simulink model "single_phase_grid_connected_inverter"  (R2022b)
settings: Solver=FixedStepDiscrete  StartTime=0.0  StopTime=0.5  FixedStep=1e-6  RelTol=1e-3
libraries: spsSeriesRLCBranchLib x9, spsFourierLib x8, spsMosfetLib x4, spsCurrentMeasurementLib x3, simulink x3, spsVoltageMeasurementLib x3, spsMeanLib x2, spsRMSLib x2, spsDCVoltageSourceLib x1, spsIdealSwitchLib x1, spspowerguiLib x1, spsControlledVoltageSourceLib x1
(part 1 of 2)
settings Model: Creator=XIAO  LastModifiedBy=XIAO
settings SolverCC: AutoInsertRateTranBlk=on
settings DataIOCC: ReturnWorkspaceOutputs=off  LoggingToFile=on

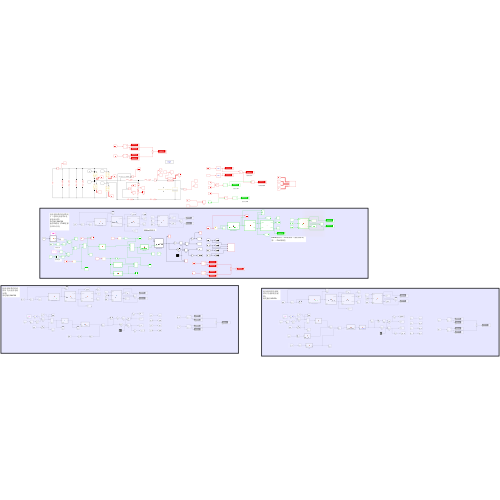
[thumbnail: Simulink's stored preview of the top-level diagram]
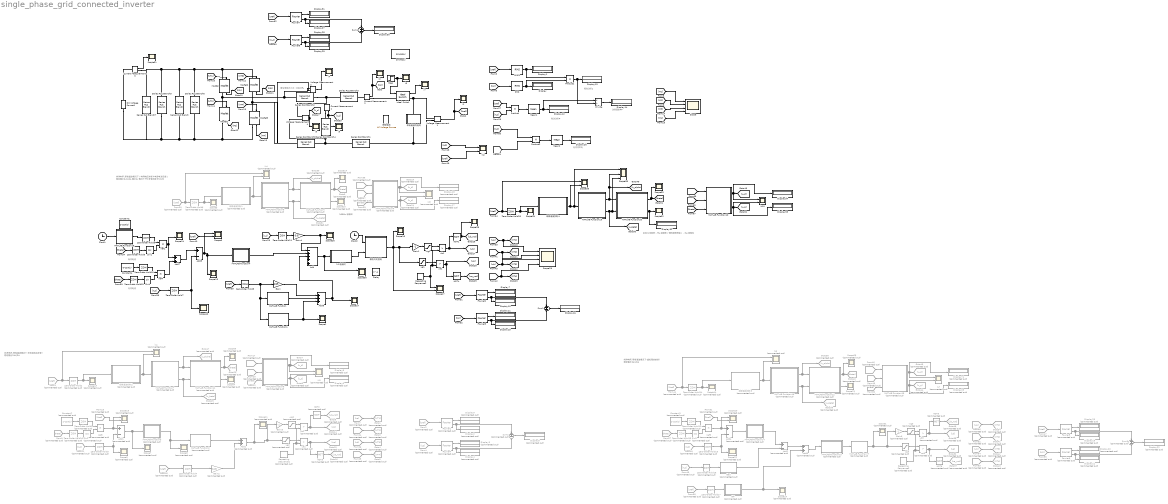
== system single_phase_grid_connected_inverter ==
  note: 100khz锁相环
  note: 视在功率s
  note: 寄生电阻大小为：R=2πfL
  note: 有功功率P
  note: 功率因数PF
  note: 纯净电网/带有谐波情况下（电网电压前馈+电容电流反馈）
      | 稳定输出24V/2A
      | 输出1A情况下THD任保持在5％以内
  note: 纯净电网/带有谐波情况下(无电容电流反馈)
      | 稳定输出24V/2A
  note: 纯净电网/带有谐波情况下(虚拟阻抗前馈)
      | 稳定输出24V/2A
  note: 无功功率Q
  note: 有功电流
  note: 无功电流
  note: 20khz锁相环，FLL锁频率（预防频率畸变），PLL锁相位
  -ug1 : Saturate  UpperLimit=1  LowerLimit=-1
  -ug2 : Saturate  Commented=on  UpperLimit=1  LowerLimit=-1
  -ug3 : Saturate  Commented=on  UpperLimit=1  LowerLimit=-1
  1.5倍延时 : MATLAB Function  TreatAsAtomicUnit=on
  Add : Sum  Inputs=-++++
  Add1 : Sum  Commented=on  Inputs=+-
  Add2 : Sum  Commented=on
  Add3 : Sum  Inputs=+-
  Add4 : Sum  Commented=on  Inputs=+-
  Add5 : Sum  Commented=on  Inputs=+-
  Add6 : Sum  Commented=on
  Add7 : Sum
  Add8 : Sum  Inputs=+++
  Clock1 : Clock
  Clock2 : Clock
  Constant1 : Constant  Value=2*sqrt(2)
  Constant2 : Constant  Commented=on  Value=2*sqrt(2)
  Constant3 : Constant  Commented=on  Value=2*sqrt(2)
  Constant4 : Constant  Value=0*sqrt(2)
  Current Measurement1 : spsCurrentMeasurementLib/Current Measurement  PhasorSimulation=off  OutputType=Complex  PSBequivalent=0
  Current Measurement2 : spsCurrentMeasurementLib/Current Measurement  PhasorSimulation=off  OutputType=Complex  PSBequivalent=0
  Current Measurement3 : spsCurrentMeasurementLib/Current Measurement  PhasorSimulation=off  OutputType=Complex  PSBequivalent=0
  DC Voltage Source1 : spsDCVoltageSourceLib/DC Voltage Source  Amplitude=45  Measurements=None
  Delay : Delay  DelayLength=1  SampleTime=5e-5
  Display{,1,7,10..16,26..34} (19 alike) : Display
  Display{2..6,8..9,17..25} (16 alike) : Display  Commented=on
  Divide : Product  Inputs=*/
  Fourier{1,4..6} (4 alike) : spsFourierLib/Fourier  Commented=on  Freq=50  n=1  InInit=[0, 0]  Ts=1e-6
  Fourier{2..3,7..8} (4 alike) : spsFourierLib/Fourier  Freq=50  n=1  InInit=[0, 0]  Ts=1e-6
  From{1..2,16,23,30,44,47,51,58} (9 alike) : From  Commented=on  GotoTag=Uref
  From17 : From  Commented=on  GotoTag=u_alpha
  From20 : From  Commented=on  GotoTag=u_beta
  From{4,21,45,49,55} (5 alike) : From  Commented=on  GotoTag=IL2
  From{9,22,39,50,57} (5 alike) : From  Commented=on  GotoTag=theta
  From24 : From  Commented=on  GotoTag=ua_not
  From25 : From  Commented=on  GotoTag=ub_not
  From26 : From  Commented=on  GotoTag=ub
  From36 : From  Commented=on  GotoTag=u_alpha
  From37 : From  Commented=on  GotoTag=u_beta
  From46 : From  Commented=on  GotoTag=u_alpha
  From48 : From  Commented=on  GotoTag=u_beta
  From52 : From  Commented=on  GotoTag=ua_not
  From53 : From  Commented=on  GotoTag=ub_not
  From54 : From  Commented=on  GotoTag=ub
  From56 : From  Commented=on  GotoTag=ua
  From7 : From  Commented=on  GotoTag=ua
  Gad : MATLAB Function  Commented=on  TreatAsAtomicUnit=on
  Gain : Gain  Gain=1/45
  Gain1 : Gain  Gain=-1
  Gain2 : Gain  Commented=on  Gain=1/45
  Gain3 : Gain  Commented=on  Gain=-1
  Gain4 : Gain  Gain=0.07
  Gain6 : Gain  Commented=on  Gain=-1
  Gff : MATLAB Function  Commented=on  TreatAsAtomicUnit=on
  Goto1 : Goto  Commented=on  GotoTag=VT1
  Goto14 : Goto  Commented=on  GotoTag=ub
  Goto15 : Goto  Commented=on  GotoTag=ua
  Goto16 : Goto  Commented=on  GotoTag=ua_not
  Goto17 : Goto  Commented=on  GotoTag=u_alpha
  Goto19 : Goto  Commented=on  GotoTag=u_beta
  Goto20 : Goto  Commented=on  GotoTag=theta
  Goto24 : Goto  Commented=on  GotoTag=u_q
  Goto25 : Goto  Commented=on  GotoTag=u_d
  Goto3 : Goto  Commented=on  GotoTag=VT2
  Goto30 : Goto  Commented=on  GotoTag=u_alpha
  Goto31 : Goto  Commented=on  GotoTag=u_beta
  Goto34 : Goto  Commented=on  GotoTag=VT1
  Goto35 : Goto  Commented=on  GotoTag=ub
  Goto36 : Goto  Commented=on  GotoTag=ua
  Goto37 : Goto  Commented=on  GotoTag=ua_not
  Goto38 : Goto  Commented=on  GotoTag=u_alpha
  Goto39 : Goto  Commented=on  GotoTag=u_beta
  Goto4 : Goto  Commented=on  GotoTag=VT3
  Goto40 : Goto  Commented=on  GotoTag=theta
  Goto41 : Goto  Commented=on  GotoTag=VT2
  Goto42 : Goto  Commented=on  GotoTag=VT3
  Goto43 : Goto  Commented=on  GotoTag=VT4
  Goto44 : Goto  Commented=on  GotoTag=u_q
  Goto45 : Goto  Commented=on  GotoTag=u_d
  Goto46 : Goto  Commented=on  GotoTag=ub_not
  Goto5 : Goto  Commented=on  GotoTag=VT4
  Goto6 : Goto  Commented=on  GotoTag=u_q
  Goto7 : Goto  Commented=on  GotoTag=u_d
  Goto8 : Goto  Commented=on  GotoTag=ub_not
  Goto9 : Goto  Commented=on  GotoTag=theta
  Ideal Switch : spsIdealSwitchLib/Ideal Switch  Ron=0.001  Lon=0  IC=0  Rs=1e5  Cs=inf  Measurements=on
  Iref1 : Product
  Iref2 : Product  Commented=on
  Iref3 : Product  Commented=on
  Iref4 : Product
  MATLAB Function : MATLAB Function  TreatAsAtomicUnit=on
  MATLAB Function1 : MATLAB Function  TreatAsAtomicUnit=on
  MATLAB Function10 : MATLAB Function  TreatAsAtomicUnit=on
  MATLAB Function11 : MATLAB Function  Commented=on  TreatAsAtomicUnit=on
  MATLAB Function12 : MATLAB Function  Commented=on  TreatAsAtomicUnit=on
  MATLAB Function13 : MATLAB Function  Commented=on  TreatAsAtomicUnit=on
  MATLAB Function14 : MATLAB Function  Commented=on  TreatAsAtomicUnit=on
  MATLAB Function15 : MATLAB Function  Commented=on  TreatAsAtomicUnit=on
  MATLAB Function16 : MATLAB Function  Commented=on  TreatAsAtomicUnit=on
  MATLAB Function17 : MATLAB Function  Commented=on  TreatAsAtomicUnit=on
  MATLAB Function18 : MATLAB Function  TreatAsAtomicUnit=on
  MATLAB Function19 : MATLAB Function  TreatAsAtomicUnit=on
  MATLAB Function2 : MATLAB Function  Commented=on  TreatAsAtomicUnit=on
  MATLAB Function20 : MATLAB Function  TreatAsAtomicUnit=on
  MATLAB Function3 : MATLAB Function  Commented=on  TreatAsAtomicUnit=on
  MATLAB Function4 : MATLAB Function  TreatAsAtomicUnit=on
  MATLAB Function5 : MATLAB Function  Commented=on  TreatAsAtomicUnit=on
  MATLAB Function6 : MATLAB Function  Commented=on  TreatAsAtomicUnit=on
  MATLAB Function7 : MATLAB Function  Commented=on  TreatAsAtomicUnit=on
  MATLAB Function8 : MATLAB Function  Commented=on  TreatAsAtomicUnit=on
  MATLAB Function9 : MATLAB Function  Commented=on  TreatAsAtomicUnit=on
  Mean1 : spsMeanLib/Mean  Freq=50  Vinit=0  Ts=5e-5
  Mean2 : spsMeanLib/Mean  Freq=50  Vinit=0  Ts=5e-5
  Mosfet{,1..3} (4 alike) : spsMosfetLib/Mosfet  Ron=0.1  Lon=0  Rd=0.01  Vfd=0  IC=0  Rs=1e5  Cs=inf  Measurements=on
  NOT1 : Logic  Operator=NOT  IconShape=distinctive  AllPortsSameDT=off  OutDataTypeStr=boolean
  NOT{2..3,5..6} (4 alike) : Logic  Commented=on  Operator=NOT  IconShape=distinctive  AllPortsSameDT=off  OutDataTypeStr=boolean
  NOT4 : Logic  Operator=NOT  IconShape=distinctive  AllPortsSameDT=off  OutDataTypeStr=boolean
  Product : Product
  Product1 : Product
  Product2 : Product
  RMS : spsRMSLib/RMS  TrueRMS=on  Freq=50  RMSInit=24  Ts=1e-6
  RMS1 : spsRMSLib/RMS  TrueRMS=on  Freq=50  RMSInit=24  Ts=1e-6
  Repeating Sequence1 : simulink/Sources/Repeating Sequence  Commented=on  rep_seq_t=[0, 5e-5, 1e-4]  rep_seq_y=[-1, 1, -1]
  Repeating Sequence2 : simulink/Sources/Repeating Sequence  rep_seq_t=[0, 5e-5, 1e-4]  rep_seq_y=[-1, 1, -1]
  Repeating Sequence3 : simulink/Sources/Repeating Sequence  Commented=on  rep_seq_t=[0, 5e-5, 1e-4]  rep_seq_y=[-1, 1, -1]
  Scope : Scope  NumInputPorts=4
  Scope{1,12..13,16,26..28,31..34} (11 alike) : Scope
  Scope{2..5,7..11,14..15,18,21..22,25} (15 alike) : Scope  Commented=on
  Scope{6,17,24,30,35} (5 alike) : Scope  NumInputPorts=2
  Scope19 : Scope  Commented=on  NumInputPorts=2
  Scope20 : Scope  Commented=on  NumInputPorts=2
  Scope23 : Scope  Commented=on  NumInputPorts=2
  Scope29 : Scope  NumInputPorts=4
  Scope36 : Scope  NumInputPorts=3
  Series RLC Branch{,5..7} (4 alike) : spsSeriesRLCBranchLib/Series RLC Branch  LConnTagsString=__new0  RConnTagsString=__new0  BranchType=RC  Resistance=0.01  Inductance=0  SetiL0=off  InitialCurrent=0  Capacitance=470e-6  Setx0=off  InitialVoltage=0  Measurements=None
  Series RLC Branch1 : spsSeriesRLCBranchLib/Series RLC Branch  LConnTagsString=__new0  RConnTagsString=__new0  BranchType=RL  Resistance=0.1  Inductance=0.00012  SetiL0=off  InitialCurrent=0  Capacitance=220e-6  Setx0=off  InitialVoltage=0  Measurements=None
  Series RLC Branch2 : spsSeriesRLCBranchLib/Series RLC Branch  LConnTagsString=__new0  RConnTagsString=__new0  BranchType=RL  Resistance=0.1  Inductance=0.0015  SetiL0=off  InitialCurrent=0  Capacitance=220e-6  Setx0=off  InitialVoltage=0  Measurements=None
  Series RLC Branch3 : spsSeriesRLCBranchLib/Series RLC Branch  LConnTagsString=__new0  RConnTagsString=__new0  BranchType=RL  Resistance=0.1  Inductance=0.00012  SetiL0=off  InitialCurrent=0  Capacitance=220e-6  Setx0=off  InitialVoltage=0  Measurements=None
  Series RLC Branch4 : spsSeriesRLCBranchLib/Series RLC Branch  LConnTagsString=__new0  RConnTagsString=__new0  BranchType=RC  Resistance=0.1  Inductance=0  SetiL0=off  InitialCurrent=0  Capacitance=10e-6  Setx0=off  InitialVoltage=0  Measurements=None
  Series RLC Branch8 : spsSeriesRLCBranchLib/Series RLC Branch  LConnTagsString=__new0  RConnTagsString=__new0  BranchType=RL  Resistance=0.1  Inductance=0.0015  SetiL0=off  InitialCurrent=0  Capacitance=220e-6  Setx0=off  InitialVoltage=0  Measurements=None
  Sin1 : Trigonometry  Operator=cos
  Sin2 : Trigonometry  Commented=on  Operator=cos
  Sin3 : Trigonometry  Commented=on  Operator=cos
  Sin4 : Trigonometry
  Step : Step  Time=0.25  SampleTime=1e-6
  Sum1 : Sum  Inputs=+-
  Sum2 : Sum  Commented=on  Inputs=+-
  Sum3 : Sum  Commented=on  Inputs=+-
  Sum4 : Sum  Inputs=+-
  Voltage Measurement1 : spsVoltageMeasurementLib/Voltage Measurement  PhasorSimulation=off  OutputType=Complex  PSBequivalent=0
  Voltage Measurement2 : spsVoltageMeasurementLib/Voltage Measurement  PhasorSimulation=off  OutputType=Complex  PSBequivalent=0
  Voltage Measurement4 : spsVoltageMeasurementLib/Voltage Measurement  PhasorSimulation=off  OutputType=Complex  PSBequivalent=0
  Zero-Order Hold{1,3..4,10,12..13,15..17} (9 alike) : ZeroOrderHold  Commented=on  SampleTime=5e-5
  Zero-Order Hold{5,7..9,11,18..20} (8 alike) : ZeroOrderHold  SampleTime=5e-5
  Zero-Order Hold14 : ZeroOrderHold  Commented=on  SampleTime=1e-5
  Zero-Order Hold2 : ZeroOrderHold  Commented=on  SampleTime=1e-5
  Zero-Order Hold6 : ZeroOrderHold  Commented=on  SampleTime=1e-5
  i{1..7} (7 alike) : Scope
  iL{1,3..7} (6 alike) : Scope  Commented=on  NumInputPorts=2
  iL10 : Scope  NumInputPorts=2
  iL2 : Scope  NumInputPorts=2
  powergui : spspowerguiLib/powergui  Priority=1  SimulationMode=Discrete  SampleTime=1e-6  frequency=60  Iterations=50  frequencyindice=0  Pbase=100e6  ErrMax=1e-4  UnitsV=kV  UnitsW=MW  buscounter=0  FunctionMessages=off  echomessages=off  EnableUseOfTLC=off  CurrentSourceSwitches=off  DisableSnubberDevices=off  DisableRonSwitches=off  DisableVfSwitches=off  DisplayEquations=off  AutomaticDiscreteSolvers=off  SolverType=Tustin/Backward Euler (TBE)  Interpol=off  ExternalGateDelay=off  methode=off  Ts=100  x0status=blocks  SPID=on  SwTol=0  HookPort=off  NonlinearTolerance=1e-4  nMaxIteration=100  ContinueOnMaxIteration=off  RestoreLinks=warning  ResistiveCurrentMeasurement=off  Frange=[0:2:500]  Ylog=off  Xlog=on  ShowGrid=off  save=off  variable=ZData  structure=0  ZoomFFT=off  StartTime=0.0  cycles=1  DisplayStyle=1  fundamental=60  FreqAxis=off  MaxFrequency=1000  frequencyindicesteady=1  RmsSteady=1  display=off
  ua1 : RelationalOperator  Operator=>  OutDataTypeStr=boolean  RndMeth=Simplest  InputSameDT=off
  ua2 : RelationalOperator  Commented=on  Operator=>  OutDataTypeStr=boolean  RndMeth=Simplest  InputSameDT=off
  ua3 : RelationalOperator  Commented=on  Operator=>  OutDataTypeStr=boolean  RndMeth=Simplest  InputSameDT=off
  ub1 : RelationalOperator  Operator=>  OutDataTypeStr=boolean  RndMeth=Simplest  InputSameDT=off
  ub2 : RelationalOperator  Commented=on  Operator=>  OutDataTypeStr=boolean  RndMeth=Simplest  InputSameDT=off
  ub3 : RelationalOperator  Commented=on  Operator=>  OutDataTypeStr=boolean  RndMeth=Simplest  InputSameDT=off
  ug1 : Saturate  UpperLimit=1  LowerLimit=-1
  ug2 : Saturate  Commented=on  UpperLimit=1  LowerLimit=-1
  ug3 : Saturate  Commented=on  UpperLimit=1  LowerLimit=-1
  带有谐波的电网 : Subsystem
  模仿开关控制 : MATLAB Function  TreatAsAtomicUnit=on
  理想电网 : spsACVoltageSourceLib/AC Voltage Source  Amplitude=24*1.414  Phase=0  Frequency=50  SampleTime=0  Measurements=None  BusType=swing  Pref=10e3  Qref=0  Qmin=-inf  Qmax=+inf
  级联谐波抑制1 : MATLAB Function  Commented=on  TreatAsAtomicUnit=on
  级联谐波抑制2 : MATLAB Function  Commented=on  TreatAsAtomicUnit=on
  级联谐波抑制3 : MATLAB Function  Commented=on  TreatAsAtomicUnit=on
  级联谐波抑制4 : MATLAB Function  TreatAsAtomicUnit=on
  wires:
  [IL2] -> RMS/1
  [VT3] -> Mosfet2/1
  RMS/1 -> Product1/2, Display/1
  Mosfet3/1 -> [M4]
  [M3] -> Scope/3
  [Uref] -> RMS1/1
  Mosfet1/1 -> [M2]
  [VT2] -> Mosfet1/1
  [M2] -> Scope/2
  [VT4] -> Mosfet3/1
  [M4] -> Scope/4
  [VT1] -> Mosfet/1
  Mosfet/1 -> [M1]
  RMS1/1 -> Product1/1, Display1/1
  Mosfet2/1 -> [M3]
  [M1] -> Scope/1
  Voltage Measurement1/1 -> i1/1, [Uref]
  [IL2] -> iL2/1
  [Uref] -> iL2/2
  Current Measurement2/1 -> [IL2], i2/1
  Voltage Measurement2/1 -> i4/1
  [Uref] -> Product/1
  [IL2] -> Product/2
  Product/1 -> Mean1/1
  Mean1/1 -> Divide/1, Display12/1
  Product1/1 -> Divide/2, Display13/1
  Divide/1 -> Display14/1
  [IL2] -> Zero-Order Hold7/1
  Zero-Order Hold9/1 -> Sin1/1
  MATLAB Function9/2(qerror) -> Scope10/1
  [Uref] -> Scope6/2
  级联谐波抑制1/1(y) -> iL4/2, MATLAB Function8/1(U_in)
  Zero-Order Hold8/1 -> MATLAB Function1/1(u), MATLAB Function/1(u), Gain/1
  MATLAB Function9/1(theta) -> Scope15/1, Goto9/1
  MATLAB Function5/2(q) -> Display17/1, Goto24/1, iL5/2
  Fourier3/1 -> Display11/1
  [ua_not] -> Scope29/2, [VT2]
  [ub] -> Scope29/3, [VT3]
  Fourier3/2 -> Sum1/2, Display15/1
  [ub_not] -> Scope29/4, [VT4]
  -ug1/1 -> ub1/1
  ug1/1 -> ua1/1
  Sum1/1 -> Display16/1
  Fourier2/2 -> Display10/1, Sum1/1
  MATLAB Function8/2(deltaU_prime) -> Goto31/1, MATLAB Function9/2(u_beta)
  [IL2] -> Fourier3/1
  [Uref] -> Fourier2/1
  [Uref] -> Zero-Order Hold8/1
  Zero-Order Hold6/1 -> 级联谐波抑制1/1(u), Scope3/1
  From36/1 -> MATLAB Function5/1(alpha)
  [ua] -> Scope29/1, [VT1]
  ub1/1 -> [ub], NOT1/1
  Gain1/1 -> -ug1/1
  ua1/1 -> [ua], NOT4/1
  MATLAB Function5/1(d) -> iL5/1, Display18/1, Goto25/1
  NOT4/1 -> [ua_not]
  Sin1/1 -> Iref1/2
  MATLAB Function8/1(U_prime) -> MATLAB Function9/1(u_alpha), Goto30/1
  From30/1 -> iL4/1, Zero-Order Hold6/1
  From39/1 -> MATLAB Function5/3(theta)
  Fourier2/1 -> Display7/1
  [theta] -> Zero-Order Hold9/1
  From37/1 -> MATLAB Function5/2(beta)
  NOT1/1 -> Scope28/1, [ub_not]
  Zero-Order Hold5/1 -> Iref1/1
  Zero-Order Hold7/1 -> Add3/2, Scope12/1
  MATLAB Function3/1(y) -> MATLAB Function2/1(u), Scope8/1
  MATLAB Function7/1(U_prime) -> MATLAB Function11/1(u_alpha), Goto17/1
  Sin2/1 -> Iref2/2
  Iref2/1 -> Scope19/1, Add1/1
  NOT3/1 -> Goto16/1
  MATLAB Function6/1(d) -> iL3/1, Display8/1, Goto7/1
  ub2/1 -> Goto14/1, NOT2/1
  Gain3/1 -> -ug2/1
  From7/1 -> Goto1/1
  From2/1 -> Fourier1/1
  From17/1 -> MATLAB Function6/1(alpha)
  From16/1 -> Zero-Order Hold4/1
  From4/1 -> Fourier4/1
  From22/1 -> MATLAB Function6/3(theta)
  级联谐波抑制2/1(y) -> iL1/2, MATLAB Function7/1(U_in)
  Sum2/1 -> Display5/1
  ug2/1 -> ua2/1
  Zero-Order Hold4/1 -> Gain2/1
  From1/1 -> iL1/1, Zero-Order Hold2/1
  -ug2/1 -> ub2/1
  Fourier1/1 -> Display9/1
  Fourier4/2 -> Sum2/2, Display4/1
  Fourier1/2 -> Display2/1, Sum2/1
  From25/1 -> Goto5/1
  From26/1 -> Goto4/1
  ua2/1 -> Goto15/1, NOT3/1
  From24/1 -> Goto3/1
  MATLAB Function11/1(theta) -> Scope9/1, Goto20/1
  Repeating Sequence1/1 -> ub2/2, ua2/2
  From9/1 -> Zero-Order Hold10/1
  Fourier4/1 -> Display3/1
  Zero-Order Hold1/1 -> Iref2/1
  MATLAB Function6/2(q) -> Display6/1, Goto6/1, iL3/2
  From20/1 -> MATLAB Function6/2(beta)
  Constant2/1 -> Zero-Order Hold1/1
  MATLAB Function11/2(qerror) -> Scope4/1
  Zero-Order Hold10/1 -> Sin2/1
  MATLAB Function7/2(deltaU_prime) -> Goto19/1, MATLAB Function11/2(u_beta)
  NOT2/1 -> Goto8/1
  From21/1 -> Zero-Order Hold3/1
  Zero-Order Hold2/1 -> 级联谐波抑制2/1(u), Scope18/1
  From23/1 -> Scope19/2
  Add1/1 -> MATLAB Function3/1(u), Scope7/1
  Zero-Order Hold3/1 -> Add1/2, Scope5/1
  Current Measurement1/1 -> [I_c], i3/1
  [I_c] -> Zero-Order Hold11/1
  Zero-Order Hold11/1 -> Gain4/1
  Add2/1 -> Scope11/1, Gain3/1, ug2/1
  Gain2/1 -> Add2/2
  Gain4/1 -> Scope26/1, Add/1
  MATLAB Function/1(y) -> Add8/2
  Fourier6/2 -> Sum3/2, Display21/1
  Fourier5/1 -> Display25/1
  -ug3/1 -> ub3/1
  From44/1 -> iL6/1, Zero-Order Hold14/1
  Zero-Order Hold15/1 -> Add4/2, Scope22/1
  From51/1 -> Scope20/2
  NOT5/1 -> Goto46/1
  From49/1 -> Zero-Order Hold15/1
  MATLAB Function16/2(deltaU_prime) -> Goto39/1, MATLAB Function12/2(u_beta)
  Zero-Order Hold14/1 -> 级联谐波抑制3/1(u), Scope14/1
  Zero-Order Hold13/1 -> Sin3/1
  Constant3/1 -> Zero-Order Hold12/1
  From57/1 -> Zero-Order Hold13/1
  MATLAB Function12/2(qerror) -> Scope21/1
  Fourier5/2 -> Display19/1, Sum3/1
  From52/1 -> Goto41/1
  MATLAB Function12/1(theta) -> Scope25/1, Goto40/1
  From48/1 -> MATLAB Function15/2(beta)
  ua3/1 -> Goto36/1, NOT6/1
  Repeating Sequence3/1 -> ub3/2, ua3/2
  Iref3/1 -> Scope20/1, Add4/1
  Zero-Order Hold12/1 -> Iref3/1
  Sin3/1 -> Iref3/2
  NOT6/1 -> Goto37/1
  Sum3/1 -> Display22/1
  MATLAB Function16/1(U_prime) -> MATLAB Function12/1(u_alpha), Goto38/1
  级联谐波抑制3/1(y) -> iL6/2, MATLAB Function16/1(U_in)
  From50/1 -> MATLAB Function15/3(theta)
  From55/1 -> Fourier6/1
  From46/1 -> MATLAB Function15/1(alpha)
  From47/1 -> Fourier5/1
  From56/1 -> Goto34/1
  Gain6/1 -> -ug3/1
  Add4/1 -> MATLAB Function14/1(u)
  ub3/1 -> Goto35/1, NOT5/1
  MATLAB Function15/1(d) -> iL7/1, Display24/1, Goto45/1
  ug3/1 -> ua3/1
  MATLAB Function15/2(q) -> Display23/1, Goto44/1, iL7/2
  From53/1 -> Goto43/1
  From54/1 -> Goto42/1
  Fourier6/1 -> Display20/1
  MATLAB Function14/1(y) -> Add5/1
  From45/1 -> Zero-Order Hold16/1
  Zero-Order Hold16/1 -> Gad/1(u)
  Gff/1(y) -> Scope23/1, Add6/2
  Zero-Order Hold17/1 -> Gff/1(u)
  From58/1 -> Zero-Order Hold17/1
  MATLAB Function2/1(y) -> Add2/1
  MATLAB Function13/1(y) -> MATLAB Function17/1(u)
  Gain/1 -> Add8/1
  MATLAB Function1/1(y) -> Add8/3, Scope1/1
  MATLAB Function17/1(y) -> Gain6/1, ug3/1, Scope2/1
  Gad/1(y) -> Add5/2
  Add5/1 -> Add6/1
  Add6/1 -> MATLAB Function13/1(u)
  Sin4/1 -> Iref4/2
  [theta] -> Zero-Order Hold19/1
  Zero-Order Hold18/1 -> Iref4/1
  Constant4/1 -> Zero-Order Hold18/1
  Zero-Order Hold19/1 -> Sin4/1
  Iref1/1 -> Add7/1, Scope24/2
  Iref4/1 -> Add7/2
  Add7/1 -> Add3/1
  [IL2] -> Product2/1
  Product2/1 -> Mean2/1
  Mean2/1 -> Display26/1
  [u_beta] -> Product2/2
  Add3/1 -> Scope6/1, MATLAB Function4/1(u), Scope13/1
  Voltage Measurement4/1 -> i5/1, [V_c]
  Step/1 -> Ideal Switch/1, i6/1
  Ideal Switch/1 -> i7/1
  Clock1/1 -> MATLAB Function18/1(t)
  MATLAB Function18/1(I_amp) -> Zero-Order Hold5/1
  Add8/1 -> Add/3, Scope27/1
  Fourier7/2 -> Display27/1, Sum4/1
  [Uref] -> Fourier7/1
  Fourier7/1 -> Display31/1
  Sum4/1 -> Display30/1
  Fourier8/1 -> Display28/1
  Fourier8/2 -> Sum4/2, Display29/1
  [V_c] -> Fourier8/1
  模仿开关控制/1(mod_out) -> Scope16/1, Gain1/1, ug1/1, Scope17/2
  Clock2/1 -> 模仿开关控制/1(t)
  Repeating Sequence2/1 -> ub1/2, ua1/2, Scope17/1
  MATLAB Function4/1(y) -> Add/2
  Add/1 -> 1.5倍延时/1(u), Scope30/1
  1.5倍延时/1(y) -> 模仿开关控制/2(mod_in)
  Current Measurement3/1 -> Scope31/1
  级联谐波抑制4/1(y) -> Scope35/2, Scope36/1, MATLAB Function19/1(uin)
  [u_beta] -> MATLAB Function10/2(beta)
  [Uref] -> Scope35/1, Zero-Order Hold20/1
  MATLAB Function20/2(qerror) -> Scope32/1, Display32/1
  [u_alpha] -> MATLAB Function10/1(alpha)
  Zero-Order Hold20/1 -> 级联谐波抑制4/1(u), Scope34/1
  MATLAB Function20/1(theta) -> Scope33/1, [theta]
  MATLAB Function10/1(d) -> iL10/1, Display34/1, [u_d]
  [theta] -> MATLAB Function10/3(theta)
  MATLAB Function10/2(q) -> Display33/1, [u_q], iL10/2
  MATLAB Function19/1(alpha) -> Scope36/2, [u_alpha], MATLAB Function20/1(u_alpha)
  MATLAB Function19/2(beta) -> Scope36/3, MATLAB Function20/2(u_beta), [u_beta]
  connections:
  Mosfet1/RConn1 -- DC Voltage Source1/LConn1 -- Series RLC Branch7/RConn1 -- Series RLC Branch5/RConn1 -- Series RLC Branch/RConn1 -- Series RLC Branch6/RConn1 -- Mosfet3/RConn1
  Mosfet/LConn1 -- Current Measurement3/RConn1 -- Series RLC Branch7/LConn1 -- Series RLC Branch5/LConn1 -- Series RLC Branch/LConn1 -- Series RLC Branch6/LConn1 -- Mosfet2/LConn1
  Series RLC Branch2/RConn1 -- Voltage Measurement2/LConn1 -- Mosfet/RConn1 -- Mosfet1/LConn1
  Mosfet3/LConn1 -- Series RLC Branch8/RConn1 -- Voltage Measurement2/LConn2 -- Mosfet2/RConn1
  Series RLC Branch2/LConn1 -- Current Measurement1/LConn1 -- Voltage Measurement4/LConn1 -- Series RLC Branch3/RConn1
  Current Measurement2/LConn1 -- Series RLC Branch3/LConn1
  带有谐波的电网/RConn1 -- Voltage Measurement1/LConn1 -- Ideal Switch/RConn1
  Current Measurement1/RConn1 -- Series RLC Branch4/LConn1
  Current Measurement2/RConn1 -- Ideal Switch/LConn1
  Current Measurement3/LConn1 -- DC Voltage Source1/RConn1
  Voltage Measurement1/LConn2 -- 带有谐波的电网/LConn1 -- Series RLC Branch1/LConn1
  Series RLC Branch4/RConn1 -- Series RLC Branch8/LConn1 -- Series RLC Branch1/RConn1 -- Voltage Measurement4/LConn2

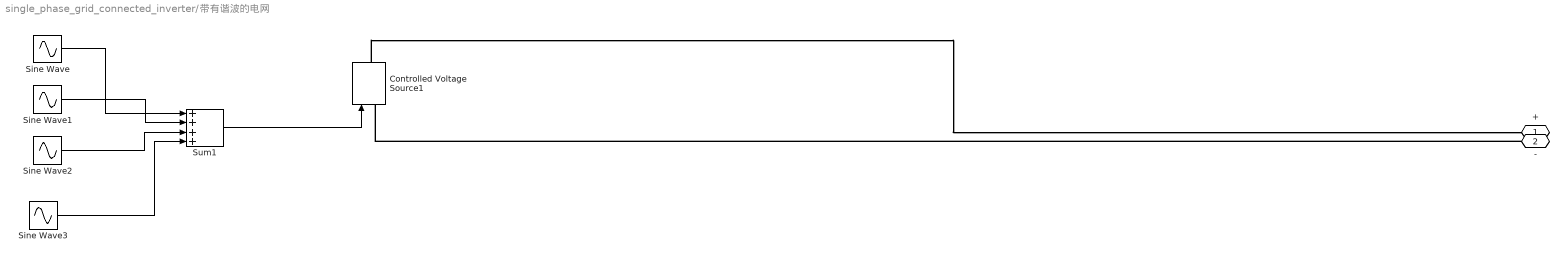
== system single_phase_grid_connected_inverter/带有谐波的电网 ==
  Controlled Voltage Source1 : spsControlledVoltageSourceLib/Controlled Voltage Source  Initialize=off  Source_Type=AC  Amplitude=0  Phase=0  Frequency=0  Measurements=Voltage
  Sine Wave : Sin  Amplitude=24*sqrt(2)  Frequency=100*pi  SampleTime=0
  Sine Wave1 : Sin  Amplitude=0.04*24*sqrt(2)  Frequency=300*pi  SampleTime=0
  Sine Wave2 : Sin  Amplitude=0.03*24*sqrt(2)  Frequency=500*pi  SampleTime=0
  Sine Wave3 : Sin  Amplitude=0.02*24*sqrt(2)  Frequency=700*pi  SampleTime=0
  Sum1 : Sum  Inputs=++++
  + : PMIOPort  Side=Right
  - : PMIOPort  Port=2  Side=Left
  wires:
  Sum1/1 -> Controlled Voltage Source1/1
  Sine Wave1/1 -> Sum1/2
  Sine Wave/1 -> Sum1/1
  Sine Wave3/1 -> Sum1/4
  Sine Wave2/1 -> Sum1/3
  connections:
  -/RConn1 -- Controlled Voltage Source1/LConn1
  Controlled Voltage Source1/RConn1 -- +/RConn1

== matlab function single_phase_grid_connected_inverter/MATLAB Function9 ==
  data: u_alpha input; theta output; u_beta input; qerror output
function [theta, qerror] = SRF_PLL(u_alpha, u_beta)
% 同步旋转坐标系锁相环 SRF-PLL（严格匹配框图逻辑）
% 输入
%   u_alpha:  α轴输入信号（对应框图的v'，与电网电压同相）
%   u_beta:   β轴输入信号（对应框图的qv'，与电网电压正交90°）
% 输出
%   theta:    锁相得到的电网相位 [0, 2π)
%   qerror:   q轴相位误差（锁相锁定时趋近于0）
% 适配：仿真步长 Ts=1e-5（10kHz采样），基波频率50Hz

    %% ===================== 1. 固定参数配置 =====================
    Ts = 1e-5;               % 采样时间，必须与全局仿真步长完全一致
    f0 = 50;                  % 电网额定基波频率 (Hz)
    w0 = 2 * pi * f0;        % 额定角频率 (rad/s)
    
    % PI控制器参数（适配10kHz采样，可按需调整）
    kp_pll = 60;              % 比例系数：增大加快锁相响应，过大易振荡
    ki_pll = 5000;            % 积分系数：增大减小稳态相位误差，过大影响稳定性

    %% ===================== 2. 持久变量初始化（仅首次运行执行） =====================
    persistent theta_prev     % 上一拍的锁相相位
    persistent xi_pll         % PI控制器的积分项（抗饱和）
    
    if isempty(theta_prev)
        theta_prev = 0;       % 相位初始值清零
        xi_pll = 0;           % 积分项初始值清零
    end

    %% ===================== 3. αβ/dq 帕克变换（核心鉴相环节） =====================
    % 标准帕克变换矩阵，严格匹配框图逻辑
    % [u_d]   = [ cosθ   sinθ ] [u_alpha]
    % [u_q]     [ -sinθ  cosθ ] [u_beta ]
    cos_theta = cos(theta_prev);
    sin_theta = sin(theta_prev);
    
    u_d = u_alpha * cos_theta + u_beta * sin_theta;  % d轴分量（对应电压幅值）
    u_q = -u_alpha * sin_theta + u_beta * cos_theta; % q轴分量（相位误差）
    
    qerror = u_q; % 输出q轴相位误差，锁相锁定时qerror→0

    %% ===================== 4. PI环路控制器 =====================
    % 位置式PI控制器，带积分抗饱和
    xi_pll = xi_pll + ki_pll * Ts * qerror;  % 积分项更新
    delta_w = kp_pll * qerror + xi_pll;      % 频率偏差量
    w_pll = w0 + delta_w;                     % 锁相得到的实时角频率

    %% ===================== 5. 积分环节（1/s）生成相位 =====================
    % 前向欧拉离散化，对应框图的1/s积分环节
    theta = theta_prev + Ts * w_pll;
    
    % 相位归一化到 [0, 2π)，防止数值溢出
    theta = mod(theta, 2 * pi);

    %% ===================== 6. 更新状态变量（为下一拍迭代准备） =====================
    theta_prev = theta;

end

== matlab function single_phase_grid_connected_inverter/级联谐波抑制1 ==
  data: u input; y output
function y = Cascade_Notch_Filter(u)
% 级联陷波滤波器：滤除3/5/7次固定频率谐波（150/250/350Hz）
% 输入u：待滤波的标量信号
% 输出y：滤波后的标量信号
% 适配：20kHz采样率（Ts=5e-5），和你的控制环完全对齐

    persistent x3_1 x3_2 x5_1 x5_2 x7_1 x7_2 first_run
    persistent b3_0 b3_1 b3_2 a3_1 a3_2
    persistent b5_0 b5_1 b5_2 a5_1 a5_2
    persistent b7_0 b7_1 b7_2 a7_1 a7_2

    %% ===================== 1. 初始化：仅首次运行 =====================
    if isempty(first_run)
        % --- 固定参数 ---
        Fs = 1e5;          % 采样频率 100kHz
        Ts = 1/Fs;            % 采样周期 5e-5s
        wc = 10;              % 截止角频率 25 rad/s
        
        % 目标谐波频率
        w3 = 2*pi*150;  % 3次谐波 150Hz
        w5 = 2*pi*250;  % 5次谐波 250Hz
        w7 = 2*pi*350;  % 7次谐波 350Hz

        % --- Tustin变换预计算系数 ---
        k = 2/Ts;
        k2 = k*k;

        % --- 3次滤波器系数 ---
        [b3_0, b3_1, b3_2, a3_1, a3_2] = calc_coeff(w3, wc, k, k2);
        % --- 5次滤波器系数 ---
        [b5_0, b5_1, b5_2, a5_1, a5_2] = calc_coeff(w5, wc, k, k2);
        % --- 7次滤波器系数 ---
        [b7_0, b7_1, b7_2, a7_1, a7_2] = calc_coeff(w7, wc, k, k2);

        % --- 显式初始化状态变量为标量 ---
        x3_1 = 0; x3_2 = 0;
        x5_1 = 0; x5_2 = 0;
        x7_1 = 0; x7_2 = 0;
        
        first_run = 1;
    end

    %% ===================== 2. 级联滤波计算（显式差分方程） =====================
    % --- 第1级：3次谐波滤波 ---
    y3 = b3_0*u + x3_1;
    x3_1_next = b3_1*u - a3_1*y3 + x3_2;
    x3_2_next = b3_2*u - a3_2*y3;
    
    % --- 第2级：5次谐波滤波 ---
    y5 = b5_0*y3 + x5_1;
    x5_1_next = b5_1*y3 - a5_1*y5 + x5_2;
    x5_2_next = b5_2*y3 - a5_2*y5;
    
    % --- 第3级：7次谐波滤波 ---
    y7 = b7_0*y5 + x7_1;
    x7_1_next = b7_1*y5 - a7_1*y7 + x7_2;
    x7_2_next = b7_2*y5 - a7_2*y7;
    
    % --- 更新状态变量 ---
    x3_1 = x3_1_next; x3_2 = x3_2_next;
    x5_1 = x5_1_next; x5_2 = x5_2_next;
    x7_1 = x7_1_next; x7_2 = x7_2_next;
    
    % --- 最终输出 ---
    y = y7;

end

%% ===================== 局部函数：预计算滤波器系数 =====================
function [b0, b1, b2, a1, a2] = calc_coeff(wn, wc, k, k2)
    % 连续域：G(s) = (s^2 + wn^2) / (s^2 + 2*wc*s + wn^2)
    % Tustin离散化：s = k*(z-1)/(z+1)
    
    % 连续域系数
    num_b0 = 1; num_b1 = 0; num_b2 = wn^2;
    den_a0 = 1; den_a1 = 2*wc; den_a2 = wn^2;
    
    % 离散化计算
    B0 = num_b0*k2 + num_b1*k + num_b2;
    B1 = 2*num_b2 - 2*num_b0*k2;
    B2 = num_b0*k2 - num_b1*k + num_b2;
    
    A0 = den_a0*k2 + den_a1*k + den_a2;
    A1 = 2*den_a2 - 2*den_a0*k2;
    A2 = den_a0*k2 - den_a1*k + den_a2;
    
    % 归一化（a0=1）
    b0 = B0 / A0;
    b1 = B1 / A0;
    b2 = B2 / A0;
    a1 = A1 / A0;
    a2 = A2 / A0;
end

== matlab function single_phase_grid_connected_inverter/级联谐波抑制2 ==
  data: u input; y output
function y = Cascade_Notch_Filter(u)
% 级联陷波滤波器：滤除3/5/7次固定频率谐波（150/250/350Hz）
% 输入u：待滤波的标量信号
% 输出y：滤波后的标量信号
% 适配：20kHz采样率（Ts=5e-5），和你的控制环完全对齐

    persistent x3_1 x3_2 x5_1 x5_2 x7_1 x7_2 first_run
    persistent b3_0 b3_1 b3_2 a3_1 a3_2
    persistent b5_0 b5_1 b5_2 a5_1 a5_2
    persistent b7_0 b7_1 b7_2 a7_1 a7_2

    %% ===================== 1. 初始化：仅首次运行 =====================
    if isempty(first_run)
        % --- 固定参数 ---
        Fs = 1e5;          % 采样频率 100kHz
        Ts = 1/Fs;            % 采样周期 5e-5s
        wc = 10;              % 截止角频率 25 rad/s
        
        % 目标谐波频率
        w3 = 2*pi*150;  % 3次谐波 150Hz
        w5 = 2*pi*250;  % 5次谐波 250Hz
        w7 = 2*pi*350;  % 7次谐波 350Hz

        % --- Tustin变换预计算系数 ---
        k = 2/Ts;
        k2 = k*k;

        % --- 3次滤波器系数 ---
        [b3_0, b3_1, b3_2, a3_1, a3_2] = calc_coeff(w3, wc, k, k2);
        % --- 5次滤波器系数 ---
        [b5_0, b5_1, b5_2, a5_1, a5_2] = calc_coeff(w5, wc, k, k2);
        % --- 7次滤波器系数 ---
        [b7_0, b7_1, b7_2, a7_1, a7_2] = calc_coeff(w7, wc, k, k2);

        % --- 显式初始化状态变量为标量 ---
        x3_1 = 0; x3_2 = 0;
        x5_1 = 0; x5_2 = 0;
        x7_1 = 0; x7_2 = 0;
        
        first_run = 1;
    end

    %% ===================== 2. 级联滤波计算（显式差分方程） =====================
    % --- 第1级：3次谐波滤波 ---
    y3 = b3_0*u + x3_1;
    x3_1_next = b3_1*u - a3_1*y3 + x3_2;
    x3_2_next = b3_2*u - a3_2*y3;
    
    % --- 第2级：5次谐波滤波 ---
    y5 = b5_0*y3 + x5_1;
    x5_1_next = b5_1*y3 - a5_1*y5 + x5_2;
    x5_2_next = b5_2*y3 - a5_2*y5;
    
    % --- 第3级：7次谐波滤波 ---
    y7 = b7_0*y5 + x7_1;
    x7_1_next = b7_1*y5 - a7_1*y7 + x7_2;
    x7_2_next = b7_2*y5 - a7_2*y7;
    
    % --- 更新状态变量 ---
    x3_1 = x3_1_next; x3_2 = x3_2_next;
    x5_1 = x5_1_next; x5_2 = x5_2_next;
    x7_1 = x7_1_next; x7_2 = x7_2_next;
    
    % --- 最终输出 ---
    y = y7;

end

%% ===================== 局部函数：预计算滤波器系数 =====================
function [b0, b1, b2, a1, a2] = calc_coeff(wn, wc, k, k2)
    % 连续域：G(s) = (s^2 + wn^2) / (s^2 + 2*wc*s + wn^2)
    % Tustin离散化：s = k*(z-1)/(z+1)
    
    % 连续域系数
    num_b0 = 1; num_b1 = 0; num_b2 = wn^2;
    den_a0 = 1; den_a1 = 2*wc; den_a2 = wn^2;
    
    % 离散化计算
    B0 = num_b0*k2 + num_b1*k + num_b2;
    B1 = 2*num_b2 - 2*num_b0*k2;
    B2 = num_b0*k2 - num_b1*k + num_b2;
    
    A0 = den_a0*k2 + den_a1*k + den_a2;
    A1 = 2*den_a2 - 2*den_a0*k2;
    A2 = den_a0*k2 - den_a1*k + den_a2;
    
    % 归一化（a0=1）
    b0 = B0 / A0;
    b1 = B1 / A0;
    b2 = B2 / A0;
    a1 = A1 / A0;
    a2 = A2 / A0;
end

== matlab function single_phase_grid_connected_inverter/MATLAB Function12 ==
  data: u_alpha input; theta output; u_beta input; qerror output
function [theta, qerror] = SRF_PLL(u_alpha, u_beta)
% 同步旋转坐标系锁相环 SRF-PLL（严格匹配框图逻辑）
% 输入
%   u_alpha:  α轴输入信号（对应框图的v'，与电网电压同相）
%   u_beta:   β轴输入信号（对应框图的qv'，与电网电压正交90°）
% 输出
%   theta:    锁相得到的电网相位 [0, 2π)
%   qerror:   q轴相位误差（锁相锁定时趋近于0）
% 适配：仿真步长 Ts=1e-5（10kHz采样），基波频率50Hz

    %% ===================== 1. 固定参数配置 =====================
    Ts = 1e-5;               % 采样时间，必须与全局仿真步长完全一致
    f0 = 50;                  % 电网额定基波频率 (Hz)
    w0 = 2 * pi * f0;        % 额定角频率 (rad/s)
    
    % PI控制器参数（适配10kHz采样，可按需调整）
    kp_pll = 60;              % 比例系数：增大加快锁相响应，过大易振荡
    ki_pll = 5000;            % 积分系数：增大减小稳态相位误差，过大影响稳定性

    %% ===================== 2. 持久变量初始化（仅首次运行执行） =====================
    persistent theta_prev     % 上一拍的锁相相位
    persistent xi_pll         % PI控制器的积分项（抗饱和）
    
    if isempty(theta_prev)
        theta_prev = 0;       % 相位初始值清零
        xi_pll = 0;           % 积分项初始值清零
    end

    %% ===================== 3. αβ/dq 帕克变换（核心鉴相环节） =====================
    % 标准帕克变换矩阵，严格匹配框图逻辑
    % [u_d]   = [ cosθ   sinθ ] [u_alpha]
    % [u_q]     [ -sinθ  cosθ ] [u_beta ]
    cos_theta = cos(theta_prev);
    sin_theta = sin(theta_prev);
    
    u_d = u_alpha * cos_theta + u_beta * sin_theta;  % d轴分量（对应电压幅值）
    u_q = -u_alpha * sin_theta + u_beta * cos_theta; % q轴分量（相位误差）
    
    qerror = u_q; % 输出q轴相位误差，锁相锁定时qerror→0

    %% ===================== 4. PI环路控制器 =====================
    % 位置式PI控制器，带积分抗饱和
    xi_pll = xi_pll + ki_pll * Ts * qerror;  % 积分项更新
    delta_w = kp_pll * qerror + xi_pll;      % 频率偏差量
    w_pll = w0 + delta_w;                     % 锁相得到的实时角频率

    %% ===================== 5. 积分环节（1/s）生成相位 =====================
    % 前向欧拉离散化，对应框图的1/s积分环节
    theta = theta_prev + Ts * w_pll;
    
    % 相位归一化到 [0, 2π)，防止数值溢出
    theta = mod(theta, 2 * pi);

    %% ===================== 6. 更新状态变量（为下一拍迭代准备） =====================
    theta_prev = theta;

end

== matlab function single_phase_grid_connected_inverter/MATLAB Function1 ==
  data: u input; y output
function y = GridVoltageFeedforward_Deriv_Module(u)
%#codegen
% 图中模块：G(s) = (L1*C/Kpwm) * s² （等效二阶微分替代，通过截止频率Hz设置ωs）
% 离散化：完整二阶系统双线性变换，工业级稳定，无数值爆炸
% 输入u：电网电压采样值 vg（单标量）
% 输出y：模块输出信号（单标量）

%% ===================== 1. 系统参数定义 =====================
L1 = 1.2e-3;         % 逆变侧电感，H
C = 10e-6;           % 滤波电容，F
k_pwm = 45;          % PWM桥臂增益
Ts = 1/20000;        % 采样周期，s（20kHz）
f_cutoff = 1150;     % 二阶低通截止频率，Hz（原7000rad/s对应≈1114Hz，可直接修改此值）
omega_s = 2 * pi * f_cutoff;  % 自动计算角频率ωs，rad/s
zeta = 0.707;        % 阻尼系数（Butterworth，无谐振峰）

%% ===================== 2. 双线性变换系数计算（完整二阶系统） =====================
a = 2 / Ts;  % 双线性变换核心系数
K = (L1 * C) / k_pwm;  % 模块基础比例系数

% --- 分子系数（修复笔误：统一使用num0，而非A0） ---
num2 = K * (omega_s^2) * (a^2);
num1 = -2 * num2;
num0 = num2;

% --- 分母系数 ---
den2 = a^2 + 2 * zeta * omega_s * a + omega_s^2;
den1 = -2 * a^2 + 2 * omega_s^2;
den0 = a^2 - 2 * zeta * omega_s * a + omega_s^2;

%% ===================== 3. 状态变量初始化 =====================
persistent u_prev1 u_prev2 y_prev1 y_prev2;
if isempty(u_prev1)
    u_prev1 = 0; % u(k-1)
    u_prev2 = 0; % u(k-2)
    y_prev1 = 0; % y(k-1)
    y_prev2 = 0; % y(k-2)
end

%% ===================== 4. 差分方程实现（修复变量名一致性） =====================
num_part = num2 * u + num1 * u_prev1 + num0 * u_prev2; % 修复：num0而非A0
den_part = den1 * y_prev1 + den0 * y_prev2;
y = (num_part - den_part) / den2;

%% ===================== 5. 更新状态变量 =====================
u_prev2 = u_prev1;
u_prev1 = u;
y_prev2 = y_prev1;
y_prev1 = y;

end

== matlab function single_phase_grid_connected_inverter/MATLAB Function13 ==
  data: u input; y output
function y = SecondOrderPadeDelay_1p5Ts(u)
% 二阶Padé逼近1.5Ts延迟模块（直接从闭环仿真提取，已验证直流增益=1）
% 输入：u - 待延迟的信号（如PR控制器输出）
% 输出：y - 延迟后的信号
% 适配：与你的闭环仿真参数100%匹配，直流增益严格等于1

persistent u_prev1 u_prev2 y_prev1 y_prev2 first_run

%% 初始化：仅首次运行
if isempty(first_run)
    % 初始化状态变量（二阶需要2个历史输入+2个历史输出）
    u_prev1 = 0;
    u_prev2 = 0;
    y_prev1 = 0;
    y_prev2 = 0;
    
    first_run = true;
end

%% 【核心】直接从闭环仿真提取的系数（已验证直流增益=1）
b0 = 0.076923076923077;
b1 = 0.153846153846154;
b2 = 1.000000000000000;
a1 = -0.153846153846154;
a2 = -0.076923076923077;

%% 二阶离散差分方程计算延迟输出
y = b0*u + b1*u_prev1 + b2*u_prev2 ...
    + a1*y_prev1 + a2*y_prev2;

%% 更新状态变量（供下一时刻使用）
u_prev2 = u_prev1;
u_prev1 = u;
y_prev2 = y_prev1;
y_prev1 = y;
end

== matlab function single_phase_grid_connected_inverter/MATLAB Function14 ==
  settings: updateMethod=DISCRETE
  data: u input; y output
function y = PR_Controller(u)
% 准谐振PR控制器，和你的.m文件1:1完全匹配
% 输入u：误差信号 error = Iref - iL2
% 输出y：PR控制器输出的调制波

persistent x_prev1 x_prev2 y_prev1 y_prev2 first_run

%% 1. 固定参数（和.m文件完全一致，无任何修改）
Ts = 5e-5;           % 采样时间 (s)，20kHz控制环
Kp = 0.2;          % PR比例系数
Kr = 20;             % PR谐振系数
w0 = 2*pi*50;        % 基波角频率 (50Hz)，和.m文件写法完全对齐
wi = pi;             % PR谐振带宽

%% 2. 初始化状态变量（仅首次运行，和.m文件初始值一致）
if isempty(first_run)
    x_prev1 = 0;  % 对应.m文件的x1_pr：上一时刻的误差
    x_prev2 = 0;  % 对应.m文件的x2_pr：上两时刻的误差
    y_prev1 = 0;  % 对应.m文件的y1_pr：上一时刻的输出
    y_prev2 = 0;  % 对应.m文件的y2_pr：上两时刻的输出
    first_run = true;
end

%% 3. 离散化系数计算（和.m文件公式、参数完全一致）
a0_pr = 4 + 2*wi*Ts + w0^2*Ts^2;
a1_pr = 2*w0^2*Ts^2 - 8;
a2_pr = 4 - 2*wi*Ts + w0^2*Ts^2;

b0_pr = 4*Kp + 4*Kp*wi*Ts + 4*Kr*wi*Ts + Kp*w0^2*Ts^2;
b1_pr = 2*Kp*w0^2*Ts^2 - 8*Kp;
b2_pr = 4*Kp - 4*Kp*wi*Ts - 4*Kr*wi*Ts + Kp*w0^2*Ts^2;

%% 4. 差分方程计算输出（和.m文件公式完全一致，符号无错误）
y = (b0_pr*u + b1_pr*x_prev1 + b2_pr*x_prev2 ...
    - a1_pr*y_prev1 - a2_pr*y_prev2) / a0_pr;

%% 5. 输出限幅（和.m文件完全一致，[-1,1]）
MODULATION_MAX = 1;
MODULATION_MIN = -1;
y = max(min(y, MODULATION_MAX), MODULATION_MIN);

%% 6. 更新状态变量（和.m文件执行顺序完全一致：先算输出→再限幅→最后更新）
x_prev2 = x_prev1;
x_prev1 = u;
y_prev2 = y_prev1;
y_prev1 = y;

end

== matlab function single_phase_grid_connected_inverter/MATLAB Function15 ==
  data: alpha input; d output; beta input; theta input; q output
function [d, q] = Park_Transform(alpha, beta, theta)
% Park变换模块（直接输入SOGI-FLL的theta，无内部积分）
% 输入：
%   alpha - α轴分量（SOGI-FLL的U_prime）
%   beta  - β轴分量（SOGI-FLL的deltaU_prime）
%   theta - 瞬时相位（SOGI-FLL直接输出的theta）
% 输出：
%   d         - d轴（直轴）分量
%   q         - q轴（交轴）分量
%   cos_theta - 相位θ的余弦值（新增输出）
%   sin_theta - 相位θ的正弦值（新增输出）

%% 核心计算
cos_theta = cos(theta);  % 相位θ的余弦值
sin_theta = sin(theta);  % 相位θ的正弦值


% 修正后的 Park 变换公式（d轴对齐同相分量 beta）
d =  alpha * cos_theta + beta * sin_theta;
q = -alpha * sin_theta + beta * cos_theta;
end

== matlab function single_phase_grid_connected_inverter/MATLAB Function16 ==
  settings: updateMethod=DISCRETE
  data: U_in input; U_prime output; deltaU_prime output
function [U_prime, deltaU_prime] = SOGI_FLL_Process(U_in)
% SOGI-FLL for Simulink: 逐点更新，内置相位积分，维护状态记忆
% 输入：U_in   - 当前时刻输入电压（标量）
% 输出：U_prime      - α轴同相输出（标量）
%       deltaU_prime - β轴正交输出（标量）
%       omega0       - 当前角频率（rad/s，标量）
%       theta        - 积分得到的瞬时相位（rad，标量，θ=∫ωdt）

%% 固定参数
dt = 1e-5;               % 仿真步长，必须与Simulink求解器步长一致
K = 1.414;               % SOGI增益
K1 = 0.25;               % 直流消除器增益
gamma = 20;              % FLL增益（你已调至46，加快收敛）
omega0_init = 100*pi;    % 初始角频率（50Hz）
w_max = 2*pi*60;         % 频率上限（60Hz）
w_min = 2*pi*40;         % 频率下限（40Hz）

%% 状态变量持久化（Simulink中必须用persistent）
persistent x1_prev x2_prev x3_prev omega0_prev theta_prev first_run

if isempty(first_run)
    % 首次运行初始化
    x1_prev = 0;
    x2_prev = 0;
    x3_prev = 0;
    omega0_prev = omega0_init;
    theta_prev = 0;       % 相位积分初始值（θ₀=0，匹配输入无初相）
    first_run = false;
end

%% 1. 计算状态导数（逐点，无矩阵）
A11 = -K1 * omega0_prev; A12 = -K1 * omega0_prev; A13 = 0;
A21 = -K  * omega0_prev; A22 = -K  * omega0_prev; A23 = -omega0_prev^2;
A31 = 0;                  A32 = 1;                   A33 = 0;

B1 = K1 * omega0_prev;
B2 = K  * omega0_prev;
B3 = 0;

dx1dt = A11*x1_prev + A12*x2_prev + A13*x3_prev + B1*U_in;
dx2dt = A21*x1_prev + A22*x2_prev + A23*x3_prev + B2*U_in;
dx3dt = A31*x1_prev + A32*x2_prev + A33*x3_prev + B3*U_in;

%% 2. 前向欧拉更新状态
x1_curr = x1_prev + dt * dx1dt;
x2_curr = x2_prev + dt * dx2dt;
x3_curr = x3_prev + dt * dx3dt;

%% 3. FLL频率更新
deltaU = U_in - x1_curr - x2_curr;
deltaU_prime_k = omega0_prev * x3_curr;
epsilon_f = deltaU * deltaU_prime_k;
domega0dt = -gamma * epsilon_f;
omega0_curr = omega0_prev + dt * domega0dt;

% 频率限幅
omega0_curr = max(min(omega0_curr, w_max), w_min);

%% 4. 内置相位积分（梯形积分，精度更高）
% 梯形积分：theta = theta_prev + (当前ω + 前一时刻ω) * dt / 2
theta_curr = theta_prev + (omega0_curr + omega0_prev) * dt / 2;
% 相位归一化（限制在[-π, π]，避免数值溢出）
theta_curr = mod(theta_curr + pi, 2*pi) - pi;

%% 5. 输出
U_prime = x2_curr;
deltaU_prime = omega0_prev * x3_curr;  % 用前一时刻ω₀计算正交分量
omega0 = omega0_curr;
theta = theta_curr;  % 新增相位输出

%% 6. 更新状态，供下一时刻使用
x1_prev = x1_curr;
x2_prev = x2_curr;
x3_prev = x3_curr;
omega0_prev = omega0_curr;
theta_prev = theta_curr;  % 更新相位状态
end

== matlab function single_phase_grid_connected_inverter/级联谐波抑制3 ==
  data: u input; y output
function y = Cascade_Notch_Filter(u)
% 级联陷波滤波器：滤除3/5/7次固定频率谐波（150/250/350Hz）
% 输入u：待滤波的标量信号
% 输出y：滤波后的标量信号
% 适配：20kHz采样率（Ts=5e-5），和你的控制环完全对齐

    persistent x3_1 x3_2 x5_1 x5_2 x7_1 x7_2 first_run
    persistent b3_0 b3_1 b3_2 a3_1 a3_2
    persistent b5_0 b5_1 b5_2 a5_1 a5_2
    persistent b7_0 b7_1 b7_2 a7_1 a7_2

    %% ===================== 1. 初始化：仅首次运行 =====================
    if isempty(first_run)
        % --- 固定参数 ---
        Fs = 1e5;          % 采样频率 100kHz
        Ts = 1/Fs;            % 采样周期 5e-5s
        wc = 10;              % 截止角频率 25 rad/s
        
        % 目标谐波频率
        w3 = 2*pi*150;  % 3次谐波 150Hz
        w5 = 2*pi*250;  % 5次谐波 250Hz
        w7 = 2*pi*350;  % 7次谐波 350Hz

        % --- Tustin变换预计算系数 ---
        k = 2/Ts;
        k2 = k*k;

        % --- 3次滤波器系数 ---
        [b3_0, b3_1, b3_2, a3_1, a3_2] = calc_coeff(w3, wc, k, k2);
        % --- 5次滤波器系数 ---
        [b5_0, b5_1, b5_2, a5_1, a5_2] = calc_coeff(w5, wc, k, k2);
        % --- 7次滤波器系数 ---
        [b7_0, b7_1, b7_2, a7_1, a7_2] = calc_coeff(w7, wc, k, k2);

        % --- 显式初始化状态变量为标量 ---
        x3_1 = 0; x3_2 = 0;
        x5_1 = 0; x5_2 = 0;
        x7_1 = 0; x7_2 = 0;
        
        first_run = 1;
    end

    %% ===================== 2. 级联滤波计算（显式差分方程） =====================
    % --- 第1级：3次谐波滤波 ---
    y3 = b3_0*u + x3_1;
    x3_1_next = b3_1*u - a3_1*y3 + x3_2;
    x3_2_next = b3_2*u - a3_2*y3;
    
    % --- 第2级：5次谐波滤波 ---
    y5 = b5_0*y3 + x5_1;
    x5_1_next = b5_1*y3 - a5_1*y5 + x5_2;
    x5_2_next = b5_2*y3 - a5_2*y5;
    
    % --- 第3级：7次谐波滤波 ---
    y7 = b7_0*y5 + x7_1;
    x7_1_next = b7_1*y5 - a7_1*y7 + x7_2;
    x7_2_next = b7_2*y5 - a7_2*y7;
    
    % --- 更新状态变量 ---
    x3_1 = x3_1_next; x3_2 = x3_2_next;
    x5_1 = x5_1_next; x5_2 = x5_2_next;
    x7_1 = x7_1_next; x7_2 = x7_2_next;
    
    % --- 最终输出 ---
    y = y7;

end

%% ===================== 局部函数：预计算滤波器系数 =====================
function [b0, b1, b2, a1, a2] = calc_coeff(wn, wc, k, k2)
    % 连续域：G(s) = (s^2 + wn^2) / (s^2 + 2*wc*s + wn^2)
    % Tustin离散化：s = k*(z-1)/(z+1)
    
    % 连续域系数
    num_b0 = 1; num_b1 = 0; num_b2 = wn^2;
    den_a0 = 1; den_a1 = 2*wc; den_a2 = wn^2;
    
    % 离散化计算
    B0 = num_b0*k2 + num_b1*k + num_b2;
    B1 = 2*num_b2 - 2*num_b0*k2;
    B2 = num_b0*k2 - num_b1*k + num_b2;
    
    A0 = den_a0*k2 + den_a1*k + den_a2;
    A1 = 2*den_a2 - 2*den_a0*k2;
    A2 = den_a0*k2 - den_a1*k + den_a2;
    
    % 归一化（a0=1）
    b0 = B0 / A0;
    b1 = B1 / A0;
    b2 = B2 / A0;
    a1 = A1 / A0;
    a2 = A2 / A0;
end

== matlab function single_phase_grid_connected_inverter/MATLAB Function17 ==
  data: u input; y output
function y = DelayCompensator(u)
%#codegen
% 延时补偿器
% 传递函数：G_com(z) = z / (m*z + (1 - m))
% 差分方程推导：
%   Y(z)*(m*z + 1 - m) = U(z)*z
%   m*z*Y(z) + (1 - m)*Y(z) = z*U(z)
%   m*y(k+1) + (1 - m)*y(k) = u(k+1)
%   改写为当前时刻形式：y(k) = [u(k) - (1 - m)*y(k-1)] / m
% 输入u：待补偿的信号（单标量）
% 输出y：补偿后的信号（单标量）

%% 1. 参数定义
m = 0.8;  % 补偿器参数，m=0.8时可完全抵消系统延时
A_limit = 10;  % 输出限幅（可按系统需求调整）

%% 2. 状态变量初始化（保存上一拍输出 y(k-1)）
persistent y_prev;
if isempty(y_prev)
    y_prev = 0;
end

%% 3. 差分方程实现（严格匹配公式推导）
% y(k) = [u(k) - (1 - m)*y(k-1)] / m
y_temp = (u - (1 - m) * y_prev) / m;

%% 4. 工程化限幅（防止数值溢出）
y = max(min(y_temp, A_limit), -A_limit);

%% 5. 更新状态变量（推进时间步）
y_prev = y_temp;
end

== matlab function single_phase_grid_connected_inverter/Gff ==
  data: u input; y output
function y = GridVoltageFeedforward_Gff_Equiv(u)
%#codegen
% 电网电压前馈 G_ff 最终正确版（完整二阶系统双线性变换，无发散）
% 连续域公式：G_ff = 1/kpwm + (L1*C/kpwm) * (ωs² s²)/(s² + 2ζωs s + ωs²)
% 离散化：完整传递函数双线性变换，无数值爆炸
% 输入u：电网电压采样值 vg（单标量）
% 输出y：G_ff前馈补偿信号（单标量）

%% ===================== 1. 系统参数定义 =====================
L1 = 1.2e-3;         % 逆变侧电感，H
C = 10e-6;           % 滤波电容，F
k_pwm = 45;          % PWM桥臂增益
Ts = 1/20000;        % 采样周期，s（20kHz）
omega_s = 7000;      % 转折角频率，rad/s
zeta = 0.707;        % 阻尼系数

%% ===================== 2. 双线性变换系数计算 =====================
a = 2 / Ts;
K_prop = 1 / k_pwm;                % 比例项系数
K_deriv = (L1 * C) / k_pwm;        % 微分项系数

% --- 等效二阶微分的离散系数 ---
num2 = K_deriv * (omega_s^2) * (a^2);
num1 = -2 * num2;
num0 = num2;
den2 = a^2 + 2 * zeta * omega_s * a + omega_s^2;
den1 = -2 * a^2 + 2 * omega_s^2;
den0 = a^2 - 2 * zeta * omega_s * a + omega_s^2;

%% ===================== 3. 状态变量初始化 =====================
persistent u_prev1 u_prev2 y_prev1 y_prev2;
if isempty(u_prev1)
    u_prev1 = 0; % u(k-1)
    u_prev2 = 0; % u(k-2)
    y_prev1 = 0; % y(k-1)
    y_prev2 = 0; % y(k-2)
end

%% ===================== 4. 差分方程实现 =====================
% 1) 比例项
term_prop = u * K_prop;
% 2) 等效二阶微分项
num_part = num2 * u + num1 * u_prev1 + num0 * u_prev2;
den_part = den1 * y_prev1 + den0 * y_prev2;
term_deriv = (num_part - den_part) / den2;
% 3) 总输出
y = term_prop + term_deriv;

%% ===================== 5. 更新状态变量 =====================
u_prev2 = u_prev1;
u_prev1 = u;
y_prev2 = y_prev1;
y_prev1 = term_deriv;

end

== matlab function single_phase_grid_connected_inverter/Gad ==
  data: u input; y output
function y = GridVoltageFeedforward_Gad_Full(u)
%#codegen
% 电网电压前馈 G_ad 最终正确版（完整二阶系统双线性变换，无发散）
% 连续域公式：G_ad(s) = (L1L2/(kPWM*Rv)) * (ωs² s²)/(s² + 2ζωs s + ωs²)
% 离散化：完整传递函数双线性变换，工业级成熟方法，无数值爆炸
% 输入u：电网电压采样值 vg（单标量）
% 输出y：G_ad前馈补偿信号（单标量）

%% ===================== 1. 系统参数定义 =====================
% 滤波器与控制参数（完全匹配你的系统）
L1 = 1.2e-3;         % 逆变侧电感，H
L2 = 120e-6;         % 网侧电感，H
k_pwm = 45;          % PWM桥臂增益
Rv = 10;             % 虚拟电阻，Ω
Ts = 1/20000;        % 采样周期，s（20kHz）
omega_s = 7000;      % 转折角频率，rad/s（1kHz，可修改为40000）
zeta = 0.707;        % 阻尼系数（Butterworth，无谐振峰）

%% ===================== 2. 双线性变换系数计算（正确完整推导） =====================
a = 2 / Ts;  % 双线性变换核心系数
K = (L1 * L2) / (k_pwm * Rv);  % G_ad基础比例系数

% --- 分子系数（完整离散化，无拆分） ---
num2 = K * (omega_s^2) * (a^2);
num1 = -2 * num2;
num0 = num2;

% --- 分母系数（完整离散化，核心：抵消分子放大） ---
den2 = a^2 + 2 * zeta * omega_s * a + omega_s^2;
den1 = -2 * a^2 + 2 * omega_s^2;
den0 = a^2 - 2 * zeta * omega_s * a + omega_s^2;

%% ===================== 3. 状态变量初始化 =====================
persistent u_prev1 u_prev2 y_prev1 y_prev2;
if isempty(u_prev1)
    u_prev1 = 0; % u(k-1)
    u_prev2 = 0; % u(k-2)
    y_prev1 = 0; % y(k-1)
    y_prev2 = 0; % y(k-2)
end

%% ===================== 4. 差分方程实现（标准二阶系统离散形式） =====================
% 离散传递函数：Y(z)/U(z) = (num2 z² + num1 z + num0)/(den2 z² + den1 z + den0)
% 差分方程：y(k) = [num2*u + num1*u_prev1 + num0*u_prev2 - den1*y_prev1 - den0*y_prev2] / den2
num_part = num2 * u + num1 * u_prev1 + num0 * u_prev2;
den_part = den1 * y_prev1 + den0 * y_prev2;
y = (num_part - den_part) / den2;

%% ===================== 5. 更新状态变量 =====================
u_prev2 = u_prev1;
u_prev1 = u;
y_prev2 = y_prev1;
y_prev1 = y;

end

== matlab function single_phase_grid_connected_inverter/MATLAB Function18 ==
  data: t input; I_amp output
function I_amp = current_amp_step(t)
% 功能：0.25s前输出0，0.25s时直接阶跃到2*sqrt(2)（无斜坡）
persistent I_target t_start;
if isempty(I_target)
    I_target = 2*sqrt(2);  % 目标值：2*根号2 ≈2.828
    t_start = 0.25;        % 触发时间：0.25s（你说的2.5s应为笔误）
end

% 核心逻辑：0.25s前=0，0.25s及以后直接输出目标值
if t < t_start
    I_amp = 0;                  % 0~0.25s：输出0
else
    I_amp = I_target;           % 0.25s后：直接设定为2*sqrt(2)
end
end

== matlab function single_phase_grid_connected_inverter/模仿开关控制 ==
  data: t input; mod_out output; mod_in input
function mod_out = gate_mod_signal(t, mod_in)
% 功能：0.25s前输出0，0.25s后输出原调制波mod_in
% 输入 t: 仿真时间 (Clock模块)
% 输入 mod_in: 原始调制波信号
% 输出 mod_out: 带使能的调制波信号

t_start = 0.25; % 合闸时间

if t < t_start
    mod_out = 0;          % 合闸前强制输出0
else
    mod_out = mod_in;      % 合闸后输出原调制波
end
end

== matlab function single_phase_grid_connected_inverter/MATLAB Function ==
  data: u input; y output
function y = CapCurrentDamping(u)
%#codegen
% 电容电流反馈有源阻尼环节
% 离散化方法：双线性变换法（Tustin），fs=20kHz
% 输入u：电容电压采样值
% 输出y：有源阻尼反馈信号

%% 固定参数（和你的系统匹配）
persistent u_prev  % 上一拍的输入值 u(k-1)
persistent y_prev  % 上一拍的输出值 y(k-1)
C = 10e-6;          % 滤波电容，F
Hi1 = 0.07;          % 反馈系数
Ts = 1/20000;        % 采样周期，s

%% 初始化状态变量
if isempty(u_prev)
    u_prev = 0;
    y_prev = 0;
end

%% 双线性变换法（Tustin）实现微分
% 连续域：G(s) = C*Hi1 * s
% 双线性变换：s = (2/Ts) * (z-1)/(z+1)
% 差分方程：y(k) = -y(k-1) + (2*C*Hi1/Ts) * (u(k) - u(k-1))
K_tustin = (2 * C * Hi1) / Ts;
y = -y_prev + K_tustin * (u - u_prev);

%% 更新状态变量
u_prev = u;
y_prev = y;
end

== matlab function single_phase_grid_connected_inverter/MATLAB Function10 ==
  data: alpha input; d output; beta input; theta input; q output
function [d, q] = Park_Transform(alpha, beta, theta)
% Park变换模块（直接输入SOGI-FLL的theta，无内部积分）
% 输入：
%   alpha - α轴分量（SOGI-FLL的U_prime）
%   beta  - β轴分量（SOGI-FLL的deltaU_prime）
%   theta - 瞬时相位（SOGI-FLL直接输出的theta）
% 输出：
%   d         - d轴（直轴）分量
%   q         - q轴（交轴）分量
%   cos_theta - 相位θ的余弦值（新增输出）
%   sin_theta - 相位θ的正弦值（新增输出）

%% 核心计算
cos_theta = cos(theta);  % 相位θ的余弦值
sin_theta = sin(theta);  % 相位θ的正弦值


% 修正后的 Park 变换公式（d轴对齐同相分量 beta）
d =  alpha * cos_theta + beta * sin_theta;
q = -alpha * sin_theta + beta * cos_theta;
end

== matlab function single_phase_grid_connected_inverter/MATLAB Function19 ==
  settings: updateMethod=DISCRETE
  data: uin input; alpha output; beta output
function [alpha, beta] = SOGI_FLL_20kHz(uin)
% 严格对应你的 m 文件：20kHz 双线性 PI-FLL
% 输入：uin   单相电压
% 输出：alpha 同相输出 uα = x2
%      beta  正交输出 uβ = omega0*x3

%% 固定参数（和你的m文件完全一致）
dt = 5e-5;
K  = 1.414;
K1 = 0.25;
gamma_p =30;
gamma_i =500;
w_max = 2*pi*60;
w_min = 2*pi*40;

%% 状态持久化
persistent x1_prev x2_prev x3_prev omega0_prev U_prev integral_f first_run;
if isempty(first_run)
    x1_prev = 0;
    x2_prev = 0;
    x3_prev = 0;
    omega0_prev = 2*pi*50;
    U_prev = uin;
    integral_f = 0;
    first_run = false;
end

%% 1. 当前输入
U_curr = uin;
omega0_prev_local = omega0_prev;

%% 2. 频率预畸变
omega_pre = (2/dt) * tan(omega0_prev_local * dt / 2);

%% 3. 状态矩阵 A, B
A_mat = [
    -K1*omega_pre, -K1*omega_pre, 0;
    -K*omega_pre,  -K*omega_pre,  -omega_pre^2;
    0,              1,              0
];
B_mat = [
    K1*omega_pre;
    K*omega_pre;
    0
];

%% 4. 双线性变换
I_mat = eye(3);
M1 = I_mat - (dt/2)*A_mat;
M2 = I_mat + (dt/2)*A_mat;
U_avg = U_curr + U_prev;

x_prev_vec = [x1_prev; x2_prev; x3_prev];
x_curr_vec = M1 \ (M2 * x_prev_vec + (dt/2)*B_mat * U_avg);

x1_curr = x_curr_vec(1);
x2_curr = x_curr_vec(2);
x3_curr = x_curr_vec(3);

%% 5. PI-FLL 频率环
deltaU = U_curr - x1_curr - x2_curr;
deltaU_prime_val = omega0_prev_local * x3_curr;
epsilon_f = deltaU * deltaU_prime_val;

integral_f = integral_f + epsilon_f * dt;
domega0dt = -gamma_p * epsilon_f - gamma_i * integral_f;
omega0_curr = omega0_prev_local + dt * domega0dt;

% 频率限幅
omega0_curr = max(min(omega0_curr, w_max), w_min);

%% 6. 输出 alpha beta
alpha = x2_curr;
beta  = omega0_curr * x3_curr;

%% 7. 更新状态
x1_prev = x1_curr;
x2_prev = x2_curr;
x3_prev = x3_curr;
omega0_prev = omega0_curr;
U_prev = U_curr;

end
